simulink model "vector_sfunc_test"  (Simulink 7.4)
settings: Solver=ode45  StartTime=0.0  StopTime=10.0  RelTol=1e-3
CloseFcn:
  | rtwprivate ssgensfun ModelCloseRequest vector_sfunc_test
settings Model: Creator=robert  LastModifiedBy=robert

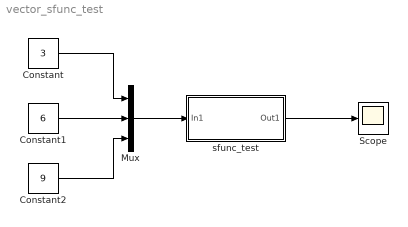
== system vector_sfunc_test ==
  Constant : Constant  Value=3  OutDataType=fixdt(1, 16)  OutScaling=2^0
  Constant1 : Constant  Value=6  OutDataType=fixdt(1, 16)  OutScaling=2^0
  Constant2 : Constant  Value=9  OutDataType=fixdt(1, 16)  OutScaling=2^0
  Mux : Mux  Inputs=3
  Scope : Scope
  sfunc_test : Subsystem
  wires:
  Constant2/1 -> Mux/3
  Constant1/1 -> Mux/2
  Constant/1 -> Mux/1
  Mux/1 -> sfunc_test/1(In1)
  sfunc_test/1(Out1) -> Scope/1

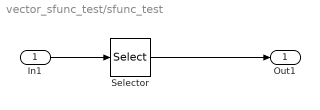
== system vector_sfunc_test/sfunc_test ==
  In1 : Inport  PortDimensions=3  OutDataType=fixdt(1, 16)  OutScaling=2^0
  Selector : Selector  InputPortWidth=3  IndexOptions=Index vector (dialog)  Indices=[3 1 2]  OutputSizes=1
  Out1 : Outport  PortDimensions=3  OutDataType=fixdt(1, 16)  OutScaling=2^0
  wires:
  In1/1 -> Selector/1
  Selector/1 -> Out1/1
